simulink model "Ex8_2"  (Simulink 6.0)
settings: Solver=ode45  StartTime=0.0  StopTime=100*Ts  RelTol=1e-3
undefined symbols (not defined in the file or in its folder): Ampl, Delta, Fin, flag, k, mism, Ts, Vref
settings Model: Creator=ivan  LastModifiedBy=Cri  ExtModeAutoUpdateStatusClock=off

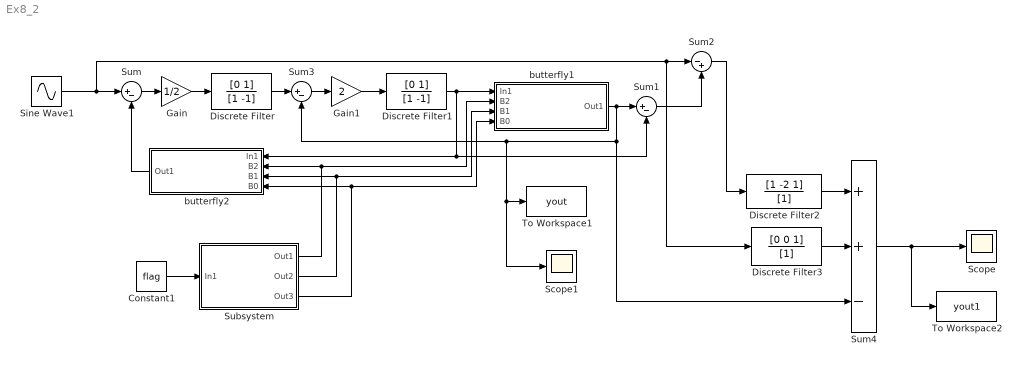
== system Ex8_2 ==
  Constant1 : Constant  Value=flag
  Discrete Filter : DiscreteFilter  Numerator=[0 1]  Denominator=[1 -1]  SampleTime=Ts
  Discrete Filter1 : DiscreteFilter  Numerator=[0 1]  Denominator=[1 -1]  SampleTime=Ts
  Discrete Filter2 : DiscreteFilter  Numerator=[1 -2 1]  Denominator=[1]  SampleTime=Ts
  Discrete Filter3 : DiscreteFilter  Numerator=[0 0 1]  Denominator=[1]  SampleTime=Ts
  Gain : Gain  Gain=1/2
  Gain1 : Gain  Gain=2
  Scope : Scope
  Scope1 : Scope
  Sine Wave1 : Sin  Amplitude=Ampl  Frequency=2*pi*Fin  SampleTime=Ts
  Subsystem : Subsystem
      mask Display:
      | color('orange');disp('BUTTERFLY\nRANDOMIZER');
      | port_label('output', 1, 'B2');
      | port_label('output', 2, 'B1');
      | port_label('output', 3, 'B0');
  Sum : Sum  Inputs=|+-
  Sum1 : Sum  Inputs=|+-
  Sum2 : Sum  Inputs=|-+
  Sum3 : Sum  Inputs=|+-
  Sum4 : Sum  Inputs=++-
  To Workspace1 : ToWorkspace  VariableName=yout  SampleTime=-1  SaveFormat=Array
  To Workspace2 : ToWorkspace  VariableName=yout1  SampleTime=-1  SaveFormat=Array
  butterfly1 : Subsystem
      mask Display:
      | disp('BUTTERFLY')
      | port_label('input', 1, 'in')
      | port_label('input', 2, 'B2')
      | port_label('input', 3, 'B1')
      | port_label('input', 4, 'B0')
      | port_label('output', 1, 'out')
  butterfly2 : Subsystem  Orientation=left
      mask Display:
      | disp('BUTTERFLY')
      | port_label('input', 1, 'in')
      | port_label('input', 2, 'B2')
      | port_label('input', 3, 'B1')
      | port_label('input', 4, 'B0')
      | port_label('output', 1, 'out')
  wires:
  Sine Wave1/1 -> Sum/1, Sum2/1, Discrete Filter3/1
  Sum/1 -> Gain/1
  Discrete Filter/1 -> Sum3/1
  Sum3/1 -> Gain1/1
  Discrete Filter1/1 -> butterfly1/1(In1), butterfly2/1(In1), Sum1/2
  Subsystem/1(Out1) -> butterfly2/2(B2), butterfly1/2(B2)
  Subsystem/2(Out2) -> butterfly2/3(B1), butterfly1/3(B1)
  Subsystem/3(Out3) -> butterfly2/4(B0), butterfly1/4(B0)
  Constant1/1 -> Subsystem/1(In1)
  Gain/1 -> Discrete Filter/1
  Gain1/1 -> Discrete Filter1/1
  butterfly2/1(Out1) -> Sum/2
  butterfly1/1(Out1) -> Sum1/1, Sum4/3, Sum3/2, To Workspace1/1, Scope1/1
  Sum1/1 -> Sum2/2
  Sum2/1 -> Discrete Filter2/1
  Discrete Filter2/1 -> Sum4/1
  Discrete Filter3/1 -> Sum4/2
  Sum4/1 -> Scope/1, To Workspace2/1

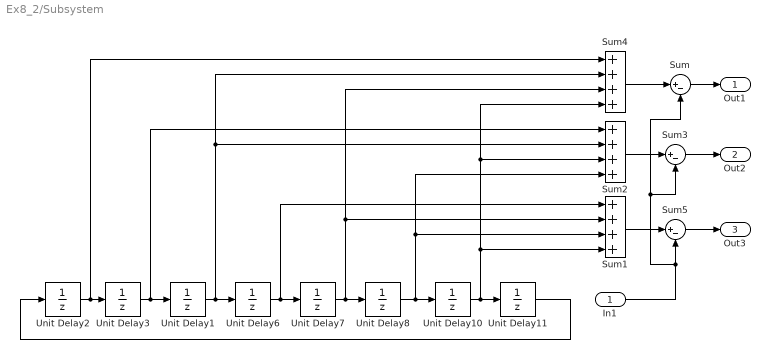
== system Ex8_2/Subsystem ==
  In1 : Inport  Port=1  LatchInput=off
  Sum : Sum  Inputs=|+-
  Sum1 : Sum  Inputs=++++
  Sum2 : Sum  Inputs=++++
  Sum3 : Sum  Inputs=|+-
  Sum4 : Sum  Inputs=++++
  Sum5 : Sum  Inputs=|+-
  Unit Delay{1,3,6..8,10..11} (7 alike) : UnitDelay  SampleTime=Ts
  Unit Delay2 : UnitDelay  X0=1  SampleTime=Ts
  Out1 : Outport
  Out2 : Outport  Port=2
  Out3 : Outport  Port=3
  wires:
  Unit Delay11/1 -> Unit Delay2/1
  Unit Delay8/1 -> Unit Delay10/1, Sum1/3, Sum2/4
  Unit Delay10/1 -> Unit Delay11/1, Sum1/4, Sum4/4, Sum2/3
  Unit Delay7/1 -> Unit Delay8/1, Sum1/2, Sum4/3
  Unit Delay2/1 -> Unit Delay3/1, Sum4/1
  Unit Delay3/1 -> Unit Delay1/1, Sum2/1
  Unit Delay1/1 -> Unit Delay6/1, Sum4/2, Sum2/2
  Unit Delay6/1 -> Unit Delay7/1, Sum1/1
  Sum/1 -> Out1/1
  Sum4/1 -> Sum/1
  Sum3/1 -> Out2/1
  Sum2/1 -> Sum3/1
  Sum1/1 -> Sum5/1
  Sum5/1 -> Out3/1
  In1/1 -> Sum5/2, Sum3/2, Sum/2

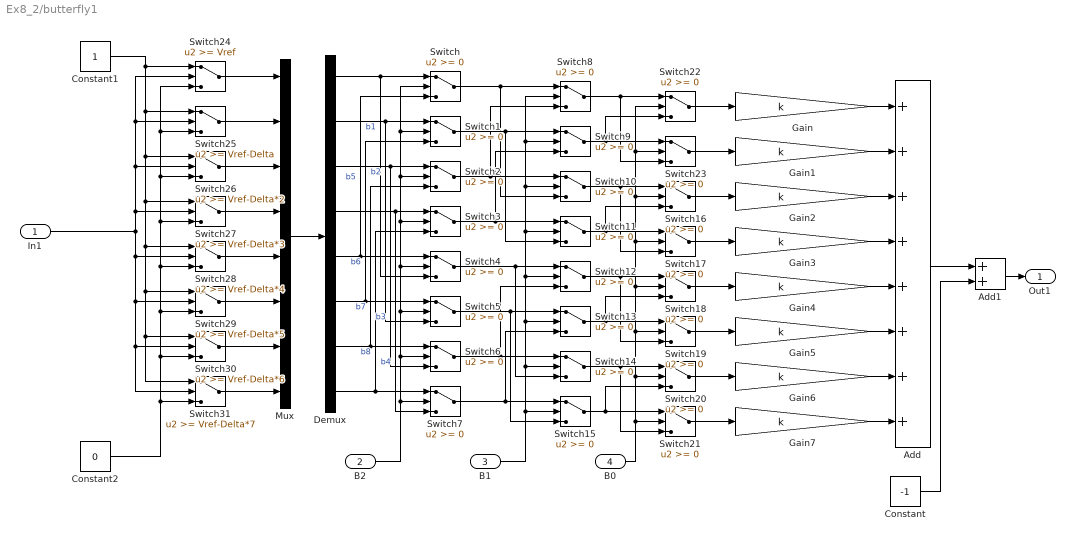
== system Ex8_2/butterfly1 ==
  In1 : Inport  Port=1  LatchInput=off
  B2 : Inport  Port=2  LatchInput=off
  B1 : Inport  Port=3  LatchInput=off
  B0 : Inport  Port=4  LatchInput=off
  Add : Sum  Inputs=++++++++  OutScaling=2^-10
  Add1 : Sum  OutScaling=2^-10
  Constant : Constant  Value=-1
  Constant1 : Constant
  Constant2 : Constant  Value=0
  Demux : Demux  Outputs=8
  Gain{,1..7} (8 alike) : Gain  Gain=k
  Mux : Mux  Inputs=8
  Switch{,1..23} (24 alike) : Switch
  Switch24 : Switch  Threshold=Vref
  Switch25 : Switch  Threshold=Vref-Delta
  Switch26 : Switch  Threshold=Vref-Delta*2
  Switch27 : Switch  Threshold=Vref-Delta*3
  Switch28 : Switch  Threshold=Vref-Delta*4
  Switch29 : Switch  Threshold=Vref-Delta*5
  Switch30 : Switch  Threshold=Vref-Delta*6
  Switch31 : Switch  Threshold=Vref-Delta*7
  Out1 : Outport
  wires:
  Demux/1 -> Switch/1, Switch4/3  "b1"
  Demux/2 -> Switch1/1, Switch5/3  "b2"
  Demux/3 -> Switch2/1, Switch6/3  "b3"
  Demux/4 -> Switch3/1, Switch7/3  "b4"
  Demux/5 -> Switch4/1, Switch/3  "b5"
  Demux/6 -> Switch5/1, Switch1/3  "b6"
  Demux/7 -> Switch6/1, Switch2/3  "b7"
  Demux/8 -> Switch7/1, Switch3/3  "b8"
  Switch/1 -> Switch10/3, Switch8/1
  Switch1/1 -> Switch9/1, Switch11/3
  Switch2/1 -> Switch10/1, Switch8/3
  Switch3/1 -> Switch11/1, Switch9/3
  Switch4/1 -> Switch12/1, Switch14/3
  Switch5/1 -> Switch13/1, Switch15/3
  Switch6/1 -> Switch14/1, Switch12/3
  Switch7/1 -> Switch15/1, Switch13/3
  Switch8/1 -> Switch22/1, Switch23/3
  Switch9/1 -> Switch23/1, Switch22/3
  Switch10/1 -> Switch16/1, Switch17/3
  Switch11/1 -> Switch17/1, Switch16/3
  Switch12/1 -> Switch18/1, Switch19/3
  Switch13/1 -> Switch19/1, Switch18/3
  Switch14/1 -> Switch20/1, Switch21/3
  Switch15/1 -> Switch21/1, Switch20/3
  Switch22/1 -> Gain/1
  Switch23/1 -> Gain1/1
  Switch16/1 -> Gain2/1
  Switch17/1 -> Gain3/1
  Switch18/1 -> Gain4/1
  Switch19/1 -> Gain5/1
  Switch20/1 -> Gain6/1
  Switch21/1 -> Gain7/1
  B2/1 -> Switch/2, Switch1/2, Switch2/2, Switch3/2, Switch4/2, Switch5/2, Switch6/2, Switch7/2
  B1/1 -> Switch15/2, Switch14/2, Switch13/2, Switch12/2, Switch11/2, Switch10/2, Switch8/2, Switch9/2
  B0/1 -> Switch22/2, Switch23/2, Switch16/2, Switch17/2, Switch18/2, Switch19/2, Switch20/2, Switch21/2
  Gain/1 -> Add/1
  Gain1/1 -> Add/2
  Gain2/1 -> Add/3
  Gain3/1 -> Add/4
  Gain4/1 -> Add/5
  Gain5/1 -> Add/6
  Gain6/1 -> Add/7
  Gain7/1 -> Add/8
  Add/1 -> Add1/1
  Constant/1 -> Add1/2
  In1/1 -> Switch24/2, Switch25/2, Switch26/2, Switch27/2, Switch28/2, Switch29/2, Switch30/2, Switch31/2
  Add1/1 -> Out1/1
  Mux/1 -> Demux/1
  Constant1/1 -> Switch24/1, Switch25/1, Switch26/1, Switch27/1, Switch28/1, Switch29/1, Switch30/1, Switch31/1
  Constant2/1 -> Switch24/3, Switch25/3, Switch26/3, Switch27/3, Switch28/3, Switch29/3, Switch30/3, Switch31/3
  Switch24/1 -> Mux/1
  Switch25/1 -> Mux/2
  Switch26/1 -> Mux/3
  Switch27/1 -> Mux/4
  Switch28/1 -> Mux/5
  Switch29/1 -> Mux/6
  Switch30/1 -> Mux/7
  Switch31/1 -> Mux/8

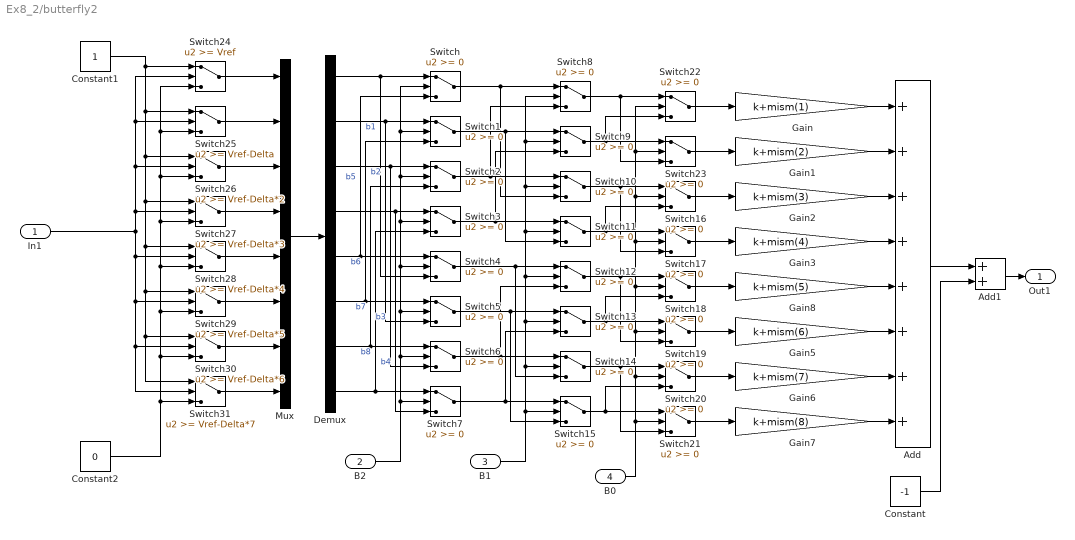
== system Ex8_2/butterfly2 ==
  In1 : Inport  Port=1  LatchInput=off
  B2 : Inport  Port=2  LatchInput=off
  B1 : Inport  Port=3  LatchInput=off
  B0 : Inport  Port=4  LatchInput=off
  Add : Sum  Inputs=++++++++  OutScaling=2^-10
  Add1 : Sum  OutScaling=2^-10
  Constant : Constant  Value=-1
  Constant1 : Constant
  Constant2 : Constant  Value=0
  Demux : Demux  Outputs=8
  Gain : Gain  Gain=k+mism(1)
  Gain1 : Gain  Gain=k+mism(2)
  Gain2 : Gain  Gain=k+mism(3)
  Gain3 : Gain  Gain=k+mism(4)
  Gain5 : Gain  Gain=k+mism(6)
  Gain6 : Gain  Gain=k+mism(7)
  Gain7 : Gain  Gain=k+mism(8)
  Gain8 : Gain  Gain=k+mism(5)
  Mux : Mux  Inputs=8
  Switch{,1..23} (24 alike) : Switch
  Switch24 : Switch  Threshold=Vref
  Switch25 : Switch  Threshold=Vref-Delta
  Switch26 : Switch  Threshold=Vref-Delta*2
  Switch27 : Switch  Threshold=Vref-Delta*3
  Switch28 : Switch  Threshold=Vref-Delta*4
  Switch29 : Switch  Threshold=Vref-Delta*5
  Switch30 : Switch  Threshold=Vref-Delta*6
  Switch31 : Switch  Threshold=Vref-Delta*7
  Out1 : Outport
  wires:
  Switch31/1 -> Mux/8
  Switch30/1 -> Mux/7
  Switch29/1 -> Mux/6
  Switch28/1 -> Mux/5
  Switch27/1 -> Mux/4
  Switch26/1 -> Mux/3
  Switch25/1 -> Mux/2
  Switch24/1 -> Mux/1
  Constant2/1 -> Switch31/3, Switch30/3, Switch29/3, Switch28/3, Switch27/3, Switch26/3, Switch25/3, Switch24/3
  Constant1/1 -> Switch31/1, Switch30/1, Switch29/1, Switch28/1, Switch27/1, Switch26/1, Switch25/1, Switch24/1
  Mux/1 -> Demux/1
  Add1/1 -> Out1/1
  In1/1 -> Switch31/2, Switch30/2, Switch29/2, Switch28/2, Switch27/2, Switch26/2, Switch25/2, Switch24/2
  Constant/1 -> Add1/2
  Add/1 -> Add1/1
  Gain7/1 -> Add/8
  Gain6/1 -> Add/7
  Gain5/1 -> Add/6
  Gain8/1 -> Add/5
  Gain3/1 -> Add/4
  Gain2/1 -> Add/3
  Gain1/1 -> Add/2
  Gain/1 -> Add/1
  B0/1 -> Switch21/2, Switch20/2, Switch19/2, Switch18/2, Switch17/2, Switch16/2, Switch23/2, Switch22/2
  B1/1 -> Switch9/2, Switch8/2, Switch10/2, Switch11/2, Switch12/2, Switch13/2, Switch14/2, Switch15/2
  B2/1 -> Switch7/2, Switch6/2, Switch5/2, Switch4/2, Switch3/2, Switch2/2, Switch1/2, Switch/2
  Switch21/1 -> Gain7/1
  Switch20/1 -> Gain6/1
  Switch19/1 -> Gain5/1
  Switch18/1 -> Gain8/1
  Switch17/1 -> Gain3/1
  Switch16/1 -> Gain2/1
  Switch23/1 -> Gain1/1
  Switch22/1 -> Gain/1
  Switch15/1 -> Switch20/3, Switch21/1
  Switch14/1 -> Switch21/3, Switch20/1
  Switch13/1 -> Switch18/3, Switch19/1
  Switch12/1 -> Switch19/3, Switch18/1
  Switch11/1 -> Switch16/3, Switch17/1
  Switch10/1 -> Switch17/3, Switch16/1
  Switch9/1 -> Switch22/3, Switch23/1
  Switch8/1 -> Switch23/3, Switch22/1
  Switch7/1 -> Switch13/3, Switch15/1
  Switch6/1 -> Switch12/3, Switch14/1
  Switch5/1 -> Switch15/3, Switch13/1
  Switch4/1 -> Switch14/3, Switch12/1
  Switch3/1 -> Switch9/3, Switch11/1
  Switch2/1 -> Switch8/3, Switch10/1
  Switch1/1 -> Switch11/3, Switch9/1
  Switch/1 -> Switch8/1, Switch10/3
  Demux/8 -> Switch3/3, Switch7/1  "b8"
  Demux/7 -> Switch2/3, Switch6/1  "b7"
  Demux/6 -> Switch1/3, Switch5/1  "b6"
  Demux/5 -> Switch/3, Switch4/1  "b5"
  Demux/4 -> Switch7/3, Switch3/1  "b4"
  Demux/3 -> Switch6/3, Switch2/1  "b3"
  Demux/2 -> Switch5/3, Switch1/1  "b2"
  Demux/1 -> Switch4/3, Switch/1  "b1"
